simulink library "ilcUpdate_cl"  (R2018b)
settings: Solver=VariableStepAuto  StartTime=0.0  StopTime=10.0  RelTol=1e-3
undefined symbols (not defined in the file): ctrl
libraries: ilcUpdateLaw_cl x1, rlsGradientEst_cl x1
settings Model: Creator=mcobb  LastModifiedBy=mcobb

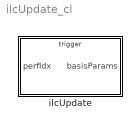
== system ilcUpdate_cl ==
  ilcUpdate : Subsystem  mask{initBasisParams=ctrl.initBasisParams.Value, lrn=ctrl.learningGain.Value, AdaptationParameter=ctrl.forgettingFactor.Value, trstRgn=ctrl.trustRegion.Value, amp=0, enableVec=ctrl.optEnable.Value}
      mask prompts: initBasisParams "Init Basis Params"; lrn "Gradient Based Learning Gain"; AdaptationParameter "Controllib:blocks:recursiveEstimationMaskAdaptationParameterFF"; trstRgn "Trust Region Dimensions"; amp "White Noise Amplitude"; enableVec "Enable Vector"
      mask TypeOptions lrn: ilcUpdateLaw/lrn
      mask TypeOptions AdaptationParameter: rlsGradientEst/AdaptationParameter
      mask TypeOptions trstRgn: ilcUpdateLaw/trstRgn
      mask TypeOptions amp: ilcUpdateLaw/amp
      mask TypeOptions enableVec: ilcUpdateLaw/enableVec
      mask DialogControl AdaptationParameter Prompt: Forgetting Factor:

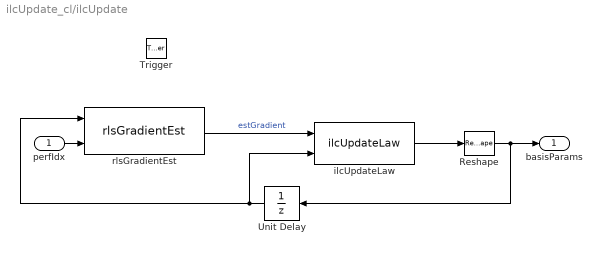
== system ilcUpdate_cl/ilcUpdate ==
  perfIdx : Inport
  Trigger : TriggerPort  VariantControl=Variant  PortDimensions=1
  Reshape : Reshape
  Unit Delay : UnitDelay  InitialCondition=[initBasisParams(:)]  SampleTime=-1
  ilcUpdateLaw : ilcUpdateLaw_cl/ilcUpdateLaw  lrn=lrn  trstRgn=trstRgn  amp=amp  enableVec=enableVec
  rlsGradientEst : rlsGradientEst_cl/rlsGradientEst  InitialParameterData=ones([2*numel(initBasisParams)+1 1])  AdaptationParameter=AdaptationParameter  Ts=1
  basisParams : Outport  InitialOutput=initBasisParams
  wires:
  rlsGradientEst/1 -> ilcUpdateLaw/1  "estGradient"
  perfIdx/1 -> rlsGradientEst/2
  ilcUpdateLaw/1 -> Reshape/1
  Unit Delay/1 -> rlsGradientEst/1, ilcUpdateLaw/2
  Reshape/1 -> Unit Delay/1, basisParams/1
